simulink model "SingleVehicle_01"  (Simulink 8.8)
settings: Solver=VariableStepAuto  StartTime=0.0  StopTime=35  RelTol=1e-3
undefined symbols (not defined in the file or in its folder): ConnectedBus, DiscIntNeverNeededParam, FromPrescan, IdealSensors, psi, x, y
undefined symbols (not defined in the file): vd
libraries: robotlib x4, PreScanUsefulBlocks x1, PreScanSimulinkLibrary x1
(part 2 of 3)

== matlab function SingleVehicle_01/Controller/CtlMainBusUnitDelayAndInit/MATLAB Function ==
  data: u input double; y output Bus: ControllerMainBus; veh_struct parameter double
function y = DelayAndInitCtlBus(u, veh_struct)
coder.extrinsic('exist')
persistent a

y0 = struct;
y0.ActuationCmdBus = struct;



y0.ActuationCmdBus.steering_cmd = 0;
y0.ActuationCmdBus.decel_cmd = 0;
y0.ActuationCmdBus.accel_cmd = 0;

y0.ArbitratedActuationReq = struct;
y0.ArbitratedActuationReq.v_des = 0;
y0.ArbitratedActuationReq.a_des = 0;
y0.ArbitratedActuationReq.psi_des = 0;
y0.ArbitratedActuationReq.dpsi_des = 0;

y0.FunctionFeatures = struct;
y0.FunctionFeatures.wpFollower = struct;
y0.FunctionFeatures.wpFollower.v_des = 0;
y0.FunctionFeatures.wpFollower.a_des = 0;
y0.FunctionFeatures.wpFollower.psi_des = 0;
y0.FunctionFeatures.wpFollower.dpsi_des = 0;

y0.situationBus = struct;
y0.situationBus.ContextualAwarenessBus = struct;
ObjectBus = struct;
ObjectBus.x = 0;
ObjectBus.y = 0;
ObjectBus.yaw = 0;
y0.situationBus.ContextualAwarenessBus.ObjectsBus = repmat(ObjectBus,100,1);
y0.situationBus.ContextualAwarenessBus.NumberObjects = 10;

y0.situationBus.wP = struct;
y0.situationBus.wP.finalWayPoint = struct;
y0.situationBus.wP.finalWayPoint.x = 0;
y0.situationBus.wP.finalWayPoint.y = 0;
y0.situationBus.wP.finalWayPoint.z = 0;
y0.situationBus.wP.finalWayPoint.treach = 0;

y0.situationBus.wP.currentWayPoint = struct;
y0.situationBus.wP.currentWayPoint.x = 0;
y0.situationBus.wP.currentWayPoint.y = 0;
y0.situationBus.wP.currentWayPoint.z = 0;
y0.situationBus.wP.currentWayPoint.treach = 0;

y0.situationBus.wP.finalWayPointIndex = uint16(1);
y0.situationBus.wP.currentWayPointIndex = uint16(10);

%y0.situationBus.wP.wayPointArray = struct;
wPArray = struct;
wPArray.x = 0;
wPArray.y = 0;
wPArray.z = 0;
wPArray.treach = 0;
y0.situationBus.wP.wayPointArray = repmat(wPArray,100,1);


y0.situationBus.selfAwarenessBus = struct;
y0.situationBus.selfAwarenessBus.x = 0;
y0.situationBus.selfAwarenessBus.y = 0;
y0.situationBus.selfAwarenessBus.z = 0;
y0.situationBus.selfAwarenessBus.theta = 0;
y0.situationBus.selfAwarenessBus.phi = 0;
y0.situationBus.selfAwarenessBus.psi = 0;
y0.situationBus.selfAwarenessBus.u = 0;
y0.situationBus.selfAwarenessBus.v = 0;
y0.situationBus.selfAwarenessBus.w = 0;
y0.situationBus.selfAwarenessBus.dtheta = 0;
y0.situationBus.selfAwarenessBus.dphi = 0;
y0.situationBus.selfAwarenessBus.dpsi = 0;

y0.IdealSensors = struct;
y0.IdealSensors.x = 0;
y0.IdealSensors.y = 0;
y0.IdealSensors.z = 0;
y0.IdealSensors.theta = 0;
y0.IdealSensors.phi = 0;
y0.IdealSensors.psi = 0;
y0.IdealSensors.u = 0;
y0.IdealSensors.v = 0;
y0.IdealSensors.w = 0;
y0.IdealSensors.dtheta = 0;
y0.IdealSensors.dphi = 0;
y0.IdealSensors.dpsi = 0;

y0.FromPrescan = struct;
y0.FromPrescan.x = 0;
y0.FromPrescan.y = 0;
y0.FromPrescan.z = 0;
y0.FromPrescan.Rotx = 0;
y0.FromPrescan.Roty = 0;
y0.FromPrescan.Rotz = 0;
y0.FromPrescan.GPS_lat = 0;
y0.FromPrescan.GPS_long = 0;
y0.FromPrescan.u = 0;
y0.FromPrescan.GPS_alt = 0;
y0.FromPrescan.heading = 0;
y0.FromPrescan.Yaw_rate = 0;


y0.ConnectedBus = struct;
ObjectBus.x = 0;
ObjectBus.y = 0;
ObjectBus.yaw = 0;
y0.ConnectedBus.ObjectsBus = repmat(ObjectBus,100,1);
y0.ConnectedBus.NumberObjects = 10;

% y1 = struct;
% y1.ActuationCmdBus = struct;
% y1.ArbitratedActuationReq = struct;
% y1.FunctionFeatures = struct;
% y1.situationBus = struct;
% y1.situationBus.situationAwarenessBus = struct;
% y1.situationBus.ContextualAwarenessBus = struct;
% y1.situationBus.wP = struct;
% y1.situationBus.wP.finalWayPoint = struct;
% y1.situationBus.wP.currentWayPoint = struct;
% y1.situationBus.selfAwarenessBus = struct;
% 
% 
% y1.ActuationCmdBus.steering_cmd = 0;
% y1.ActuationCmdBus.decel_cmd = 0;
% y1.ActuationCmdBus.accel_cmd = 0;
% 
% y1.ArbitratedActuationReq.v_des = 0;
% y1.ArbitratedActuationReq.a_des = 0;
% y1.ArbitratedActuationReq.psi_des = 0;
% y1.ArbitratedActuationReq.dpsi_des = 0;
% 
% y1.FunctionFeatures.wpFollower = struct;
% y1.FunctionFeatures.wpFollower.v_des = 0;
% y1.FunctionFeatures.wpFollower.a_des = 0;
% y1.FunctionFeatures.wpFollower.psi_des = 0;
% y1.FunctionFeatures.wpFollower.dpsi_des = 0;
% 
% %y1.situationBus.ContextualAwarenessBus.ObjectsBus = struct;
% ObjectBus = struct;
% ObjectBus.x = 0;
% ObjectBus.y = 0;
% ObjectBus.yaw = 0;
% 
% y1.situationBus.ContextualAwarenessBus.ObjectsBus = repmat(ObjectBus,100,1);
% y1.situationBus.ContextualAwarenessBus.ObjectsBus(1, 1).x = 0;
% y1.situationBus.ContextualAwarenessBus.ObjectsBus(1, 1).y = 0;
% y1.situationBus.ContextualAwarenessBus.ObjectsBus(1, 1).yaw = 0;
% y1.situationBus.ContextualAwarenessBus.ObjectsBus(2, 1).x = 0;
% y1.situationBus.ContextualAwarenessBus.ObjectsBus(2, 1).y = 0;
% y1.situationBus.ContextualAwarenessBus.ObjectsBus(2, 1).yaw = 0;
% y1.situationBus.ContextualAwarenessBus.ObjectsBus(3, 1).x = 0;
% y1.situationBus.ContextualAwarenessBus.ObjectsBus(3, 1).y = 0;
% y1.situationBus.ContextualAwarenessBus.ObjectsBus(3, 1).yaw = 0;
% y1.situationBus.ContextualAwarenessBus.ObjectsBus(4, 1).x = 0;
% y1.situationBus.ContextualAwarenessBus.ObjectsBus(4, 1).y = 0;
% y1.situationBus.ContextualAwarenessBus.ObjectsBus(4, 1).yaw = 0;
% y1.situationBus.ContextualAwarenessBus.ObjectsBus(5, 1).x = 0;
% y1.situationBus.ContextualAwarenessBus.ObjectsBus(5, 1).y = 0;
% y1.situationBus.ContextualAwarenessBus.ObjectsBus(5, 1).yaw = 0;
% y1.situationBus.ContextualAwarenessBus.ObjectsBus(6, 1).x = 0;
% y1.situationBus.ContextualAwarenessBus.ObjectsBus(6, 1).y = 0;
% y1.situationBus.ContextualAwarenessBus.ObjectsBus(6, 1).yaw = 0;
% y1.situationBus.ContextualAwarenessBus.ObjectsBus(7, 1).x = 0;
% y1.situationBus.ContextualAwarenessBus.ObjectsBus(7, 1).y = 0;
% y1.situationBus.ContextualAwarenessBus.ObjectsBus(7, 1).yaw = 0;
% y1.situationBus.ContextualAwarenessBus.ObjectsBus(8, 1).x = 0;
% y1.situationBus.ContextualAwarenessBus.ObjectsBus(8, 1).y = 0;
% y1.situationBus.ContextualAwarenessBus.ObjectsBus(8, 1).yaw = 0;
% y1.situationBus.ContextualAwarenessBus.ObjectsBus(9, 1).x = 0;
% y1.situationBus.ContextualAwarenessBus.ObjectsBus(9, 1).y = 0;
% y1.situationBus.ContextualAwarenessBus.ObjectsBus(9, 1).yaw = 0;
% y1.situationBus.ContextualAwarenessBus.ObjectsBus(10, 1).x = 0;
% y1.situationBus.ContextualAwarenessBus.ObjectsBus(10, 1).y = 0;
% y1.situationBus.ContextualAwarenessBus.ObjectsBus(10, 1).yaw = 0;
% y1.situationBus.ContextualAwarenessBus.ObjectsBus(11, 1).x = 0;
% y1.situationBus.ContextualAwarenessBus.ObjectsBus(11, 1).y = 0;
% y1.situationBus.ContextualAwarenessBus.ObjectsBus(11, 1).yaw = 0;
% y1.situationBus.ContextualAwarenessBus.ObjectsBus(12, 1).x = 0;
% y1.situationBus.ContextualAwarenessBus.ObjectsBus(12, 1).y = 0;
% y1.situationBus.ContextualAwarenessBus.ObjectsBus(12, 1).yaw = 0;
% y1.situationBus.ContextualAwarenessBus.ObjectsBus(13, 1).x = 0;
% y1.situationBus.ContextualAwarenessBus.ObjectsBus(13, 1).y = 0;
% y1.situationBus.ContextualAwarenessBus.ObjectsBus(13, 1).yaw = 0;
% y1.situationBus.ContextualAwarenessBus.ObjectsBus(14, 1).x = 0;
% y1.situationBus.ContextualAwarenessBus.ObjectsBus(14, 1).y = 0;
% y1.situationBus.ContextualAwarenessBus.ObjectsBus(14, 1).yaw = 0;
% y1.situationBus.ContextualAwarenessBus.ObjectsBus(15, 1).x = 0;
% y1.situationBus.ContextualAwarenessBus.ObjectsBus(15, 1).y = 0;
% y1.situationBus.ContextualAwarenessBus.ObjectsBus(15, 1).yaw = 0;
% y1.situationBus.ContextualAwarenessBus.ObjectsBus(16, 1).x = 0;
% y1.situationBus.ContextualAwarenessBus.ObjectsBus(16, 1).y = 0;
% y1.situationBus.ContextualAwarenessBus.ObjectsBus(16, 1).yaw = 0;
% y1.situationBus.ContextualAwarenessBus.ObjectsBus(17, 1).x = 0;
% y1.situationBus.ContextualAwarenessBus.ObjectsBus(17, 1).y = 0;
% y1.situationBus.ContextualAwarenessBus.ObjectsBus(17, 1).yaw = 0;
% y1.situationBus.ContextualAwarenessBus.ObjectsBus(18, 1).x = 0;
% y1.situationBus.ContextualAwarenessBus.ObjectsBus(18, 1).y = 0;
% y1.situationBus.ContextualAwarenessBus.ObjectsBus(18, 1).yaw = 0;
% y1.situationBus.ContextualAwarenessBus.ObjectsBus(19, 1).x = 0;
% y1.situationBus.ContextualAwarenessBus.ObjectsBus(19, 1).y = 0;
% y1.situationBus.ContextualAwarenessBus.ObjectsBus(19, 1).yaw = 0;
% y1.situationBus.ContextualAwarenessBus.ObjectsBus(20, 1).x = 0;
% y1.situationBus.ContextualAwarenessBus.ObjectsBus(20, 1).y = 0;
% y1.situationBus.ContextualAwarenessBus.ObjectsBus(20, 1).yaw = 0;
% y1.situationBus.ContextualAwarenessBus.ObjectsBus(21, 1).x = 0;
% y1.situationBus.ContextualAwarenessBus.ObjectsBus(21, 1).y = 0;
% y1.situationBus.ContextualAwarenessBus.ObjectsBus(21, 1).yaw = 0;
% y1.situationBus.ContextualAwarenessBus.ObjectsBus(22, 1).x = 0;
% y1.situationBus.ContextualAwarenessBus.ObjectsBus(22, 1).y = 0;
% y1.situationBus.ContextualAwarenessBus.ObjectsBus(22, 1).yaw = 0;
% y1.situationBus.ContextualAwarenessBus.ObjectsBus(23, 1).x = 0;
% y1.situationBus.ContextualAwarenessBus.ObjectsBus(23, 1).y = 0;
% y1.situationBus.ContextualAwarenessBus.ObjectsBus(23, 1).yaw = 0;
% y1.situationBus.ContextualAwarenessBus.ObjectsBus(24, 1).x = 0;
% y1.situationBus.ContextualAwarenessBus.ObjectsBus(24, 1).y = 0;
% y1.situationBus.ContextualAwarenessBus.ObjectsBus(24, 1).yaw = 0;
% y1.situationBus.ContextualAwarenessBus.ObjectsBus(25, 1).x = 0;
% y1.situationBus.ContextualAwarenessBus.ObjectsBus(25, 1).y = 0;
% y1.situationBus.ContextualAwarenessBus.ObjectsBus(25, 1).yaw = 0;
% y1.situationBus.ContextualAwarenessBus.ObjectsBus(26, 1).x = 0;
% y1.situationBus.ContextualAwarenessBus.ObjectsBus(26, 1).y = 0;
% y1.situationBus.ContextualAwarenessBus.ObjectsBus(26, 1).yaw = 0;
% y1.situationBus.ContextualAwarenessBus.ObjectsBus(27, 1).x = 0;
% y1.situationBus.ContextualAwarenessBus.ObjectsBus(27, 1).y = 0;
% y1.situationBus.ContextualAwarenessBus.ObjectsBus(27, 1).yaw = 0;
% y1.situationBus.ContextualAwarenessBus.ObjectsBus(28, 1).x = 0;
% y1.situationBus.ContextualAwarenessBus.ObjectsBus(28, 1).y = 0;
% y1.situationBus.ContextualAwarenessBus.ObjectsBus(28, 1).yaw = 0;
% y1.situationBus.ContextualAwarenessBus.ObjectsBus(29, 1).x = 0;
% y1.situationBus.ContextualAwarenessBus.ObjectsBus(29, 1).y = 0;
% y1.situationBus.ContextualAwarenessBus.ObjectsBus(29, 1).yaw = 0;
% y1.situationBus.ContextualAwarenessBus.ObjectsBus(30, 1).x = 0;
% y1.situationBus.ContextualAwarenessBus.ObjectsBus(30, 1).y = 0;
% y1.situationBus.ContextualAwarenessBus.ObjectsBus(30, 1).yaw = 0;
% y1.situationBus.ContextualAwarenessBus.ObjectsBus(31, 1).x = 0;
% y1.situationBus.ContextualAwarenessBus.ObjectsBus(31, 1).y = 0;
% y1.situationBus.ContextualAwarenessBus.ObjectsBus(31, 1).yaw = 0;
% y1.situationBus.ContextualAwarenessBus.ObjectsBus(32, 1).x = 0;
% y1.situationBus.ContextualAwarenessBus.ObjectsBus(32, 1).y = 0;
% y1.situationBus.ContextualAwarenessBus.ObjectsBus(32, 1).yaw = 0;
% y1.situationBus.ContextualAwarenessBus.ObjectsBus(33, 1).x = 0;
% y1.situationBus.ContextualAwarenessBus.ObjectsBus(33, 1).y = 0;
% y1.situationBus.ContextualAwarenessBus.ObjectsBus(33, 1).yaw = 0;
% y1.situationBus.ContextualAwarenessBus.ObjectsBus(34, 1).x = 0;
% y1.situationBus.ContextualAwarenessBus.ObjectsBus(34, 1).y = 0;
% y1.situationBus.ContextualAwarenessBus.ObjectsBus(34, 1).yaw = 0;
% y1.situationBus.ContextualAwarenessBus.ObjectsBus(35, 1).x = 0;
% y1.situationBus.ContextualAwarenessBus.ObjectsBus(35, 1).y = 0;
% y1.situationBus.ContextualAwarenessBus.ObjectsBus(35, 1).yaw = 0;
% y1.situationBus.ContextualAwarenessBus.ObjectsBus(36, 1).x = 0;
% y1.situationBus.ContextualAwarenessBus.ObjectsBus(36, 1).y = 0;
% y1.situationBus.ContextualAwarenessBus.ObjectsBus(36, 1).yaw = 0;
% y1.situationBus.ContextualAwarenessBus.ObjectsBus(37, 1).x = 0;
% y1.situationBus.ContextualAwarenessBus.ObjectsBus(37, 1).y = 0;
% y1.situationBus.ContextualAwarenessBus.ObjectsBus(37, 1).yaw = 0;
% y1.situationBus.ContextualAwarenessBus.ObjectsBus(38, 1).x = 0;
% y1.situationBus.ContextualAwarenessBus.ObjectsBus(38, 1).y = 0;
% y1.situationBus.ContextualAwarenessBus.ObjectsBus(38, 1).yaw = 0;
% y1.situationBus.ContextualAwarenessBus.ObjectsBus(39, 1).x = 0;
% y1.situationBus.ContextualAwarenessBus.ObjectsBus(39, 1).y = 0;
% y1.situationBus.ContextualAwarenessBus.ObjectsBus(39, 1).yaw = 0;
% y1.situationBus.ContextualAwarenessBus.ObjectsBus(40, 1).x = 0;
% y1.situationBus.ContextualAwarenessBus.ObjectsBus(40, 1).y = 0;
% y1.situationBus.ContextualAwarenessBus.ObjectsBus(40, 1).yaw = 0;
% y1.situationBus.ContextualAwarenessBus.ObjectsBus(41, 1).x = 0;
% y1.situationBus.ContextualAwarenessBus.ObjectsBus(41, 1).y = 0;
% y1.situationBus.ContextualAwarenessBus.ObjectsBus(41, 1).yaw = 0;
% y1.situationBus.ContextualAwarenessBus.ObjectsBus(42, 1).x = 0;
% y1.situationBus.ContextualAwarenessBus.ObjectsBus(42, 1).y = 0;
% y1.situationBus.ContextualAwarenessBus.ObjectsBus(42, 1).yaw = 0;
% y1.situationBus.ContextualAwarenessBus.ObjectsBus(43, 1).x = 0;
% y1.situationBus.ContextualAwarenessBus.ObjectsBus(43, 1).y = 0;
% y1.situationBus.ContextualAwarenessBus.ObjectsBus(43, 1).yaw = 0;
% y1.situationBus.ContextualAwarenessBus.ObjectsBus(44, 1).x = 0;
% y1.situationBus.ContextualAwarenessBus.ObjectsBus(44, 1).y = 0;
% y1.situationBus.ContextualAwarenessBus.ObjectsBus(44, 1).yaw = 0;
% y1.situationBus.ContextualAwarenessBus.ObjectsBus(45, 1).x = 0;
% y1.situationBus.ContextualAwarenessBus.ObjectsBus(45, 1).y = 0;
% y1.situationBus.ContextualAwarenessBus.ObjectsBus(45, 1).yaw = 0;
% y1.situationBus.ContextualAwarenessBus.ObjectsBus(46, 1).x = 0;
% y1.situationBus.ContextualAwarenessBus.ObjectsBus(46, 1).y = 0;
% y1.situationBus.ContextualAwarenessBus.ObjectsBus(46, 1).yaw = 0;
% y1.situationBus.ContextualAwarenessBus.ObjectsBus(47, 1).x = 0;
% y1.situationBus.ContextualAwarenessBus.ObjectsBus(47, 1).y = 0;
% y1.situationBus.ContextualAwarenessBus.ObjectsBus(47, 1).yaw = 0;
% y1.situationBus.ContextualAwarenessBus.ObjectsBus(48, 1).x = 0;
% y1.situationBus.ContextualAwarenessBus.ObjectsBus(48, 1).y = 0;
% y1.situationBus.ContextualAwarenessBus.ObjectsBus(48, 1).yaw = 0;
% y1.situationBus.ContextualAwarenessBus.ObjectsBus(49, 1).x = 0;
% y1.situationBus.ContextualAwarenessBus.ObjectsBus(49, 1).y = 0;
% y1.situationBus.ContextualAwarenessBus.ObjectsBus(49, 1).yaw = 0;
% y1.situationBus.ContextualAwarenessBus.ObjectsBus(50, 1).x = 0;
% y1.situationBus.ContextualAwarenessBus.ObjectsBus(50, 1).y = 0;
% y1.situationBus.ContextualAwarenessBus.ObjectsBus(50, 1).yaw = 0;
% y1.situationBus.ContextualAwarenessBus.ObjectsBus(51, 1).x = 0;
% y1.situationBus.ContextualAwarenessBus.ObjectsBus(51, 1).y = 0;
% y1.situationBus.ContextualAwarenessBus.ObjectsBus(51, 1).yaw = 0;
% y1.situationBus.ContextualAwarenessBus.ObjectsBus(52, 1).x = 0;
% y1.situationBus.ContextualAwarenessBus.ObjectsBus(52, 1).y = 0;
% y1.situationBus.ContextualAwarenessBus.ObjectsBus(52, 1).yaw = 0;
% y1.situationBus.ContextualAwarenessBus.ObjectsBus(53, 1).x = 0;
% y1.situationBus.ContextualAwarenessBus.ObjectsBus(53, 1).y = 0;
% y1.situationBus.ContextualAwarenessBus.ObjectsBus(53, 1).yaw = 0;
% y1.situationBus.ContextualAwarenessBus.ObjectsBus(54, 1).x = 0;
% y1.situationBus.ContextualAwarenessBus.ObjectsBus(54, 1).y = 0;
% y1.situationBus.ContextualAwarenessBus.ObjectsBus(54, 1).yaw = 0;
% y1.situationBus.ContextualAwarenessBus.ObjectsBus(55, 1).x = 0;
% y1.situationBus.ContextualAwarenessBus.ObjectsBus(55, 1).y = 0;
% y1.situationBus.ContextualAwarenessBus.ObjectsBus(55, 1).yaw = 0;
% y1.situationBus.ContextualAwarenessBus.ObjectsBus(56, 1).x = 0;
% y1.situationBus.ContextualAwarenessBus.ObjectsBus(56, 1).y = 0;
% y1.situationBus.ContextualAwarenessBus.ObjectsBus(56, 1).yaw = 0;
% y1.situationBus.ContextualAwarenessBus.ObjectsBus(57, 1).x = 0;
% y1.situationBus.ContextualAwarenessBus.ObjectsBus(57, 1).y = 0;
% y1.situationBus.ContextualAwarenessBus.ObjectsBus(57, 1).yaw = 0;
% y1.situationBus.ContextualAwarenessBus.ObjectsBus(58, 1).x = 0;
% y1.situationBus.ContextualAwarenessBus.ObjectsBus(58, 1).y = 0;
% y1.situationBus.ContextualAwarenessBus.ObjectsBus(58, 1).yaw = 0;
% y1.situationBus.ContextualAwarenessBus.ObjectsBus(59, 1).x = 0;
% y1.situationBus.ContextualAwarenessBus.ObjectsBus(59, 1).y = 0;
% y1.situationBus.ContextualAwarenessBus.ObjectsBus(59, 1).yaw = 0;
% y1.situationBus.ContextualAwarenessBus.ObjectsBus(60, 1).x = 0;
% y1.situationBus.ContextualAwarenessBus.ObjectsBus(60, 1).y = 0;
% y1.situationBus.ContextualAwarenessBus.ObjectsBus(60, 1).yaw = 0;
% y1.situationBus.ContextualAwarenessBus.ObjectsBus(61, 1).x = 0;
% y1.situationBus.ContextualAwarenessBus.ObjectsBus(61, 1).y = 0;
% y1.situationBus.ContextualAwarenessBus.ObjectsBus(61, 1).yaw = 0;
% y1.situationBus.ContextualAwarenessBus.ObjectsBus(62, 1).x = 0;
% y1.situationBus.ContextualAwarenessBus.ObjectsBus(62, 1).y = 0;
% y1.situationBus.ContextualAwarenessBus.ObjectsBus(62, 1).yaw = 0;
% y1.situationBus.ContextualAwarenessBus.ObjectsBus(63, 1).x = 0;
% y1.situationBus.ContextualAwarenessBus.ObjectsBus(63, 1).y = 0;
% y1.situationBus.ContextualAwarenessBus.ObjectsBus(63, 1).yaw = 0;
% y1.situationBus.ContextualAwarenessBus.ObjectsBus(64, 1).x = 0;
% y1.situationBus.ContextualAwarenessBus.ObjectsBus(64, 1).y = 0;
% y1.situationBus.ContextualAwarenessBus.ObjectsBus(64, 1).yaw = 0;
% y1.situationBus.ContextualAwarenessBus.ObjectsBus(65, 1).x = 0;
% y1.situationBus.ContextualAwarenessBus.ObjectsBus(65, 1).y = 0;
% y1.situationBus.ContextualAwarenessBus.ObjectsBus(65, 1).yaw = 0;
% y1.situationBus.ContextualAwarenessBus.ObjectsBus(66, 1).x = 0;
% y1.situationBus.ContextualAwarenessBus.ObjectsBus(66, 1).y = 0;
% y1.situationBus.ContextualAwarenessBus.ObjectsBus(66, 1).yaw = 0;
% y1.situationBus.ContextualAwarenessBus.ObjectsBus(67, 1).x = 0;
% y1.situationBus.ContextualAwarenessBus.ObjectsBus(67, 1).y = 0;
% y1.situationBus.ContextualAwarenessBus.ObjectsBus(67, 1).yaw = 0;
% y1.situationBus.ContextualAwarenessBus.ObjectsBus(68, 1).x = 0;
% y1.situationBus.ContextualAwarenessBus.ObjectsBus(68, 1).y = 0;
% y1.situationBus.ContextualAwarenessBus.ObjectsBus(68, 1).yaw = 0;
% y1.situationBus.ContextualAwarenessBus.ObjectsBus(69, 1).x = 0;
% y1.situationBus.ContextualAwarenessBus.ObjectsBus(69, 1).y = 0;
% y1.situationBus.ContextualAwarenessBus.ObjectsBus(69, 1).yaw = 0;
% y1.situationBus.ContextualAwarenessBus.ObjectsBus(70, 1).x = 0;
% y1.situationBus.ContextualAwarenessBus.ObjectsBus(70, 1).y = 0;
% y1.situationBus.ContextualAwarenessBus.ObjectsBus(70, 1).yaw = 0;
% y1.situationBus.ContextualAwarenessBus.ObjectsBus(71, 1).x = 0;
% y1.situationBus.ContextualAwarenessBus.ObjectsBus(71, 1).y = 0;
% y1.situationBus.ContextualAwarenessBus.ObjectsBus(71, 1).yaw = 0;
% y1.situationBus.ContextualAwarenessBus.ObjectsBus(72, 1).x = 0;
% y1.situationBus.ContextualAwarenessBus.ObjectsBus(72, 1).y = 0;
% y1.situationBus.ContextualAwarenessBus.ObjectsBus(72, 1).yaw = 0;
% y1.situationBus.ContextualAwarenessBus.ObjectsBus(73, 1).x = 0;
% y1.situationBus.ContextualAwarenessBus.ObjectsBus(73, 1).y = 0;
% y1.situationBus.ContextualAwarenessBus.ObjectsBus(73, 1).yaw = 0;
% y1.situationBus.ContextualAwarenessBus.ObjectsBus(74, 1).x = 0;
% y1.situationBus.ContextualAwarenessBus.ObjectsBus(74, 1).y = 0;
% y1.situationBus.ContextualAwarenessBus.ObjectsBus(74, 1).yaw = 0;
% y1.situationBus.ContextualAwarenessBus.ObjectsBus(75, 1).x = 0;
% y1.situationBus.ContextualAwarenessBus.ObjectsBus(75, 1).y = 0;
% y1.situationBus.ContextualAwarenessBus.ObjectsBus(75, 1).yaw = 0;
% y1.situationBus.ContextualAwarenessBus.ObjectsBus(76, 1).x = 0;
% y1.situationBus.ContextualAwarenessBus.ObjectsBus(76, 1).y = 0;
% y1.situationBus.ContextualAwarenessBus.ObjectsBus(76, 1).yaw = 0;
% y1.situationBus.ContextualAwarenessBus.ObjectsBus(77, 1).x = 0;
% y1.situationBus.ContextualAwarenessBus.ObjectsBus(77, 1).y = 0;
% y1.situationBus.ContextualAwarenessBus.ObjectsBus(77, 1).yaw = 0;
% y1.situationBus.ContextualAwarenessBus.ObjectsBus(78, 1).x = 0;
% y1.situationBus.ContextualAwarenessBus.ObjectsBus(78, 1).y = 0;
% y1.situationBus.ContextualAwarenessBus.ObjectsBus(78, 1).yaw = 0;
% y1.situationBus.ContextualAwarenessBus.ObjectsBus(79, 1).x = 0;
% y1.situationBus.ContextualAwarenessBus.ObjectsBus(79, 1).y = 0;
% y1.situationBus.ContextualAwarenessBus.ObjectsBus(79, 1).yaw = 0;
% y1.situationBus.ContextualAwarenessBus.ObjectsBus(80, 1).x = 0;
% y1.situationBus.ContextualAwarenessBus.ObjectsBus(80, 1).y = 0;
% y1.situationBus.ContextualAwarenessBus.ObjectsBus(80, 1).yaw = 0;
% y1.situationBus.ContextualAwarenessBus.ObjectsBus(81, 1).x = 0;
% y1.situationBus.ContextualAwarenessBus.ObjectsBus(81, 1).y = 0;
% y1.situationBus.ContextualAwarenessBus.ObjectsBus(81, 1).yaw = 0;
% y1.situationBus.ContextualAwarenessBus.ObjectsBus(82, 1).x = 0;
% y1.situationBus.ContextualAwarenessBus.ObjectsBus(82, 1).y = 0;
% y1.situationBus.ContextualAwarenessBus.ObjectsBus(82, 1).yaw = 0;
% y1.situationBus.ContextualAwarenessBus.ObjectsBus(83, 1).x = 0;
% y1.situationBus.ContextualAwarenessBus.ObjectsBus(83, 1).y = 0;
% y1.situationBus.ContextualAwarenessBus.ObjectsBus(83, 1).yaw = 0;
% y1.situationBus.ContextualAwarenessBus.ObjectsBus(84, 1).x = 0;
% y1.situationBus.ContextualAwarenessBus.ObjectsBus(84, 1).y = 0;
% y1.situationBus.ContextualAwarenessBus.ObjectsBus(84, 1).yaw = 0;
% y1.situationBus.ContextualAwarenessBus.ObjectsBus(85, 1).x = 0;
% y1.situationBus.ContextualAwarenessBus.ObjectsBus(85, 1).y = 0;
% y1.situationBus.ContextualAwarenessBus.ObjectsBus(85, 1).yaw = 0;
% y1.situationBus.ContextualAwarenessBus.ObjectsBus(86, 1).x = 0;
% y1.situationBus.ContextualAwarenessBus.ObjectsBus(86, 1).y = 0;
% y1.situationBus.ContextualAwarenessBus.ObjectsBus(86, 1).yaw = 0;
% y1.situationBus.ContextualAwarenessBus.ObjectsBus(87, 1).x = 0;
% y1.situationBus.ContextualAwarenessBus.ObjectsBus(87, 1).y = 0;
% y1.situationBus.ContextualAwarenessBus.ObjectsBus(87, 1).yaw = 0;
% y1.situationBus.ContextualAwarenessBus.ObjectsBus(88, 1).x = 0;
% y1.situationBus.ContextualAwarenessBus.ObjectsBus(88, 1).y = 0;
% y1.situationBus.ContextualAwarenessBus.ObjectsBus(88, 1).yaw = 0;
% y1.situationBus.ContextualAwarenessBus.ObjectsBus(89, 1).x = 0;
% y1.situationBus.ContextualAwarenessBus.ObjectsBus(89, 1).y = 0;
% y1.situationBus.ContextualAwarenessBus.ObjectsBus(89, 1).yaw = 0;
% y1.situationBus.ContextualAwarenessBus.ObjectsBus(90, 1).x = 0;
% y1.situationBus.ContextualAwarenessBus.ObjectsBus(90, 1).y = 0;
% y1.situationBus.ContextualAwarenessBus.ObjectsBus(90, 1).yaw = 0;
% y1.situationBus.ContextualAwarenessBus.ObjectsBus(91, 1).x = 0;
% y1.situationBus.ContextualAwarenessBus.ObjectsBus(91, 1).y = 0;
% y1.situationBus.ContextualAwarenessBus.ObjectsBus(91, 1).yaw = 0;
% y1.situationBus.ContextualAwarenessBus.ObjectsBus(92, 1).x = 0;
% y1.situationBus.ContextualAwarenessBus.ObjectsBus(92, 1).y = 0;
% y1.situationBus.ContextualAwarenessBus.ObjectsBus(92, 1).yaw = 0;
% y1.situationBus.ContextualAwarenessBus.ObjectsBus(93, 1).x = 0;
% y1.situationBus.ContextualAwarenessBus.ObjectsBus(93, 1).y = 0;
% y1.situationBus.ContextualAwarenessBus.ObjectsBus(93, 1).yaw = 0;
% y1.situationBus.ContextualAwarenessBus.ObjectsBus(94, 1).x = 0;
% y1.situationBus.ContextualAwarenessBus.ObjectsBus(94, 1).y = 0;
% y1.situationBus.ContextualAwarenessBus.ObjectsBus(94, 1).yaw = 0;
% y1.situationBus.ContextualAwarenessBus.ObjectsBus(95, 1).x = 0;
% y1.situationBus.ContextualAwarenessBus.ObjectsBus(95, 1).y = 0;
% y1.situationBus.ContextualAwarenessBus.ObjectsBus(95, 1).yaw = 0;
% y1.situationBus.ContextualAwarenessBus.ObjectsBus(96, 1).x = 0;
% y1.situationBus.ContextualAwarenessBus.ObjectsBus(96, 1).y = 0;
% y1.situationBus.ContextualAwarenessBus.ObjectsBus(96, 1).yaw = 0;
% y1.situationBus.ContextualAwarenessBus.ObjectsBus(97, 1).x = 0;
% y1.situationBus.ContextualAwarenessBus.ObjectsBus(97, 1).y = 0;
% y1.situationBus.ContextualAwarenessBus.ObjectsBus(97, 1).yaw = 0;
% y1.situationBus.ContextualAwarenessBus.ObjectsBus(98, 1).x = 0;
% y1.situationBus.ContextualAwarenessBus.ObjectsBus(98, 1).y = 0;
% y1.situationBus.ContextualAwarenessBus.ObjectsBus(98, 1).yaw = 0;
% y1.situationBus.ContextualAwarenessBus.ObjectsBus(99, 1).x = 0;
% y1.situationBus.ContextualAwarenessBus.ObjectsBus(99, 1).y = 0;
% y1.situationBus.ContextualAwarenessBus.ObjectsBus(99, 1).yaw = 0;
% y1.situationBus.ContextualAwarenessBus.ObjectsBus(100, 1).x = 0;
% y1.situationBus.ContextualAwarenessBus.ObjectsBus(100, 1).y = 0;
% y1.situationBus.ContextualAwarenessBus.ObjectsBus(100, 1).yaw = 0;
% y1.situationBus.ContextualAwarenessBus.NumberObjects = 0;
% 
% y1.situationBus.wP.finalWayPoint.x = 0;
% y1.situationBus.wP.finalWayPoint.y = 0;
% y1.situationBus.wP.finalWayPoint.z = 0;
% y1.situationBus.wP.finalWayPoint.treach = 0;
% 
% y1.situationBus.wP.currentWayPoint.x = 0;
% y1.situationBus.wP.currentWayPoint.y = 0;
% y1.situationBus.wP.currentWayPoint.z = 0;
% y1.situationBus.wP.currentWayPoint.treach = 0;
% y1.situationBus.wP.finalWayPointIndex = uint16(0);
% y1.situationBus.wP.currentWayPointIndex = uint16(0);
% %y1.situationBus.wP.wayPointArray = struct;
% wPpoint = struct;
% wPpoint.x = 0;
% wPpoint.y = 0;
% wPpoint.z = 0;
% wPpoint.treach = 0;
% y1.situationBus.wP.wayPointArray = repmat(wPpoint,100,1)
% y1.situationBus.wP.wayPointArray(1, 1).x = 0;
% y1.situationBus.wP.wayPointArray(1, 1).y = 0;
% y1.situationBus.wP.wayPointArray(1, 1).z = 0;
% y1.situationBus.wP.wayPointArray(1, 1).treach = 0;
% y1.situationBus.wP.wayPointArray(2, 1).x = 0;
% y1.situationBus.wP.wayPointArray(2, 1).y = 0;
% y1.situationBus.wP.wayPointArray(2, 1).z = 0;
% y1.situationBus.wP.wayPointArray(2, 1).treach = 0;
% y1.situationBus.wP.wayPointArray(3, 1).x = 0;
% y1.situationBus.wP.wayPointArray(3, 1).y = 0;
% y1.situationBus.wP.wayPointArray(3, 1).z = 0;
% y1.situationBus.wP.wayPointArray(3, 1).treach = 0;
% y1.situationBus.wP.wayPointArray(4, 1).x = 0;
% y1.situationBus.wP.wayPointArray(4, 1).y = 0;
% y1.situationBus.wP.wayPointArray(4, 1).z = 0;
% y1.situationBus.wP.wayPointArray(4, 1).treach = 0;
% y1.situationBus.wP.wayPointArray(5, 1).x = 0;
% y1.situationBus.wP.wayPointArray(5, 1).y = 0;
% y1.situationBus.wP.wayPointArray(5, 1).z = 0;
% y1.situationBus.wP.wayPointArray(5, 1).treach = 0;
% y1.situationBus.wP.wayPointArray(6, 1).x = 0;
% y1.situationBus.wP.wayPointArray(6, 1).y = 0;
% y1.situationBus.wP.wayPointArray(6, 1).z = 0;
% y1.situationBus.wP.wayPointArray(6, 1).treach = 0;
% y1.situationBus.wP.wayPointArray(7, 1).x = 0;
% y1.situationBus.wP.wayPointArray(7, 1).y = 0;
% y1.situationBus.wP.wayPointArray(7, 1).z = 0;
% y1.situationBus.wP.wayPointArray(7, 1).treach = 0;
% y1.situationBus.wP.wayPointArray(8, 1).x = 0;
% y1.situationBus.wP.wayPointArray(8, 1).y = 0;
% y1.situationBus.wP.wayPointArray(8, 1).z = 0;
% y1.situationBus.wP.wayPointArray(8, 1).treach = 0;
% y1.situationBus.wP.wayPointArray(9, 1).x = 0;
% y1.situationBus.wP.wayPointArray(9, 1).y = 0;
% y1.situationBus.wP.wayPointArray(9, 1).z = 0;
% y1.situationBus.wP.wayPointArray(9, 1).treach = 0;
% y1.situationBus.wP.wayPointArray(10, 1).x = 0;
% y1.situationBus.wP.wayPointArray(10, 1).y = 0;
% y1.situationBus.wP.wayPointArray(10, 1).z = 0;
% y1.situationBus.wP.wayPointArray(10, 1).treach = 0;
% y1.situationBus.wP.wayPointArray(11, 1).x = 0;
% y1.situationBus.wP.wayPointArray(11, 1).y = 0;
% y1.situationBus.wP.wayPointArray(11, 1).z = 0;
% y1.situationBus.wP.wayPointArray(11, 1).treach = 0;
% y1.situationBus.wP.wayPointArray(12, 1).x = 0;
% y1.situationBus.wP.wayPointArray(12, 1).y = 0;
% y1.situationBus.wP.wayPointArray(12, 1).z = 0;
% y1.situationBus.wP.wayPointArray(12, 1).treach = 0;
% y1.situationBus.wP.wayPointArray(13, 1).x = 0;
% y1.situationBus.wP.wayPointArray(13, 1).y = 0;
% y1.situationBus.wP.wayPointArray(13, 1).z = 0;
% y1.situationBus.wP.wayPointArray(13, 1).treach = 0;
% y1.situationBus.wP.wayPointArray(14, 1).x = 0;
% y1.situationBus.wP.wayPointArray(14, 1).y = 0;
% y1.situationBus.wP.wayPointArray(14, 1).z = 0;
% y1.situationBus.wP.wayPointArray(14, 1).treach = 0;
% y1.situationBus.wP.wayPointArray(15, 1).x = 0;
% y1.situationBus.wP.wayPointArray(15, 1).y = 0;
% y1.situationBus.wP.wayPointArray(15, 1).z = 0;
% y1.situationBus.wP.wayPointArray(15, 1).treach = 0;
% y1.situationBus.wP.wayPointArray(16, 1).x = 0;
% y1.situationBus.wP.wayPointArray(16, 1).y = 0;
% y1.situationBus.wP.wayPointArray(16, 1).z = 0;
% y1.situationBus.wP.wayPointArray(16, 1).treach = 0;
% y1.situationBus.wP.wayPointArray(17, 1).x = 0;
% y1.situationBus.wP.wayPointArray(17, 1).y = 0;
% y1.situationBus.wP.wayPointArray(17, 1).z = 0;
% y1.situationBus.wP.wayPointArray(17, 1).treach = 0;
% y1.situationBus.wP.wayPointArray(18, 1).x = 0;
% y1.situationBus.wP.wayPointArray(18, 1).y = 0;
% y1.situationBus.wP.wayPointArray(18, 1).z = 0;
% y1.situationBus.wP.wayPointArray(18, 1).treach = 0;
% y1.situationBus.wP.wayPointArray(19, 1).x = 0;
% y1.situationBus.wP.wayPointArray(19, 1).y = 0;
% y1.situationBus.wP.wayPointArray(19, 1).z = 0;
% y1.situationBus.wP.wayPointArray(19, 1).treach = 0;
% y1.situationBus.wP.wayPointArray(20, 1).x = 0;
% y1.situationBus.wP.wayPointArray(20, 1).y = 0;
% y1.situationBus.wP.wayPointArray(20, 1).z = 0;
% y1.situationBus.wP.wayPointArray(20, 1).treach = 0;
% y1.situationBus.wP.wayPointArray(21, 1).x = 0;
% y1.situationBus.wP.wayPointArray(21, 1).y = 0;
% y1.situationBus.wP.wayPointArray(21, 1).z = 0;
% y1.situationBus.wP.wayPointArray(21, 1).treach = 0;
% y1.situationBus.wP.wayPointArray(22, 1).x = 0;
% y1.situationBus.wP.wayPointArray(22, 1).y = 0;
% y1.situationBus.wP.wayPointArray(22, 1).z = 0;
% y1.situationBus.wP.wayPointArray(22, 1).treach = 0;
% y1.situationBus.wP.wayPointArray(23, 1).x = 0;
% y1.situationBus.wP.wayPointArray(23, 1).y = 0;
% y1.situationBus.wP.wayPointArray(23, 1).z = 0;
% y1.situationBus.wP.wayPointArray(23, 1).treach = 0;
% y1.situationBus.wP.wayPointArray(24, 1).x = 0;
% y1.situationBus.wP.wayPointArray(24, 1).y = 0;
% y1.situationBus.wP.wayPointArray(24, 1).z = 0;
% y1.situationBus.wP.wayPointArray(24, 1).treach = 0;
% y1.situationBus.wP.wayPointArray(25, 1).x = 0;
% y1.situationBus.wP.wayPointArray(25, 1).y = 0;
% y1.situationBus.wP.wayPointArray(25, 1).z = 0;
% y1.situationBus.wP.wayPointArray(25, 1).treach = 0;
% y1.situationBus.wP.wayPointArray(26, 1).x = 0;
% y1.situationBus.wP.wayPointArray(26, 1).y = 0;
% y1.situationBus.wP.wayPointArray(26, 1).z = 0;
% y1.situationBus.wP.wayPointArray(26, 1).treach = 0;
% y1.situationBus.wP.wayPointArray(27, 1).x = 0;
% y1.situationBus.wP.wayPointArray(27, 1).y = 0;
% y1.situationBus.wP.wayPointArray(27, 1).z = 0;
% y1.situationBus.wP.wayPointArray(27, 1).treach = 0;
% y1.situationBus.wP.wayPointArray(28, 1).x = 0;
% y1.situationBus.wP.wayPointArray(28, 1).y = 0;
% y1.situationBus.wP.wayPointArray(28, 1).z = 0;
% y1.situationBus.wP.wayPointArray(28, 1).treach = 0;
% y1.situationBus.wP.wayPointArray(29, 1).x = 0;
% y1.situationBus.wP.wayPointArray(29, 1).y = 0;
% y1.situationBus.wP.wayPointArray(29, 1).z = 0;
% y1.situationBus.wP.wayPointArray(29, 1).treach = 0;
% y1.situationBus.wP.wayPointArray(30, 1).x = 0;
% y1.situationBus.wP.wayPointArray(30, 1).y = 0;
% y1.situationBus.wP.wayPointArray(30, 1).z = 0;
% y1.situationBus.wP.wayPointArray(30, 1).treach = 0;
% y1.situationBus.wP.wayPointArray(31, 1).x = 0;
% y1.situationBus.wP.wayPointArray(31, 1).y = 0;
% y1.situationBus.wP.wayPointArray(31, 1).z = 0;
% y1.situationBus.wP.wayPointArray(31, 1).treach = 0;
% y1.situationBus.wP.wayPointArray(32, 1).x = 0;
% y1.situationBus.wP.wayPointArray(32, 1).y = 0;
% y1.situationBus.wP.wayPointArray(32, 1).z = 0;
% y1.situationBus.wP.wayPointArray(32, 1).treach = 0;
% y1.situationBus.wP.wayPointArray(33, 1).x = 0;
% y1.situationBus.wP.wayPointArray(33, 1).y = 0;
% y1.situationBus.wP.wayPointArray(33, 1).z = 0;
% y1.situationBus.wP.wayPointArray(33, 1).treach = 0;
% y1.situationBus.wP.wayPointArray(34, 1).x = 0;
% y1.situationBus.wP.wayPointArray(34, 1).y = 0;
% y1.situationBus.wP.wayPointArray(34, 1).z = 0;
% y1.situationBus.wP.wayPointArray(34, 1).treach = 0;
% y1.situationBus.wP.wayPointArray(35, 1).x = 0;
% y1.situationBus.wP.wayPointArray(35, 1).y = 0;
% y1.situationBus.wP.wayPointArray(35, 1).z = 0;
% y1.situationBus.wP.wayPointArray(35, 1).treach = 0;
% y1.situationBus.wP.wayPointArray(36, 1).x = 0;
% y1.situationBus.wP.wayPointArray(36, 1).y = 0;
% y1.situationBus.wP.wayPointArray(36, 1).z = 0;
% y1.situationBus.wP.wayPointArray(36, 1).treach = 0;
% y1.situationBus.wP.wayPointArray(37, 1).x = 0;
% y1.situationBus.wP.wayPointArray(37, 1).y = 0;
% y1.situationBus.wP.wayPointArray(37, 1).z = 0;
% y1.situationBus.wP.wayPointArray(37, 1).treach = 0;
% y1.situationBus.wP.wayPointArray(38, 1).x = 0;
% y1.situationBus.wP.wayPointArray(38, 1).y = 0;
% y1.situationBus.wP.wayPointArray(38, 1).z = 0;
% y1.situationBus.wP.wayPointArray(38, 1).treach = 0;
% y1.situationBus.wP.wayPointArray(39, 1).x = 0;
% y1.situationBus.wP.wayPointArray(39, 1).y = 0;
% y1.situationBus.wP.wayPointArray(39, 1).z = 0;
% y1.situationBus.wP.wayPointArray(39, 1).treach = 0;
% y1.situationBus.wP.wayPointArray(40, 1).x = 0;
% y1.situationBus.wP.wayPointArray(40, 1).y = 0;
% y1.situationBus.wP.wayPointArray(40, 1).z = 0;
% y1.situationBus.wP.wayPointArray(40, 1).treach = 0;
% y1.situationBus.wP.wayPointArray(41, 1).x = 0;
% y1.situationBus.wP.wayPointArray(41, 1).y = 0;
% y1.situationBus.wP.wayPointArray(41, 1).z = 0;
% y1.situationBus.wP.wayPointArray(41, 1).treach = 0;
% y1.situationBus.wP.wayPointArray(42, 1).x = 0;
% y1.situationBus.wP.wayPointArray(42, 1).y = 0;
% y1.situationBus.wP.wayPointArray(42, 1).z = 0;
% y1.situationBus.wP.wayPointArray(42, 1).treach = 0;
% y1.situationBus.wP.wayPointArray(43, 1).x = 0;
% y1.situationBus.wP.wayPointArray(43, 1).y = 0;
% y1.situationBus.wP.wayPointArray(43, 1).z = 0;
% y1.situationBus.wP.wayPointArray(43, 1).treach = 0;
% y1.situationBus.wP.wayPointArray(44, 1).x = 0;
% y1.situationBus.wP.wayPointArray(44, 1).y = 0;
% y1.situationBus.wP.wayPointArray(44, 1).z = 0;
% y1.situationBus.wP.wayPointArray(44, 1).treach = 0;
% y1.situationBus.wP.wayPointArray(45, 1).x = 0;
% y1.situationBus.wP.wayPointArray(45, 1).y = 0;
% y1.situationBus.wP.wayPointArray(45, 1).z = 0;
% y1.situationBus.wP.wayPointArray(45, 1).treach = 0;
% y1.situationBus.wP.wayPointArray(46, 1).x = 0;
% y1.situationBus.wP.wayPointArray(46, 1).y = 0;
% y1.situationBus.wP.wayPointArray(46, 1).z = 0;
% y1.situationBus.wP.wayPointArray(46, 1).treach = 0;
% y1.situationBus.wP.wayPointArray(47, 1).x = 0;
% y1.situationBus.wP.wayPointArray(47, 1).y = 0;
% y1.situationBus.wP.wayPointArray(47, 1).z = 0;
% y1.situationBus.wP.wayPointArray(47, 1).treach = 0;
% y1.situationBus.wP.wayPointArray(48, 1).x = 0;
% y1.situationBus.wP.wayPointArray(48, 1).y = 0;
% y1.situationBus.wP.wayPointArray(48, 1).z = 0;
% y1.situationBus.wP.wayPointArray(48, 1).treach = 0;
% y1.situationBus.wP.wayPointArray(49, 1).x = 0;
% y1.situationBus.wP.wayPointArray(49, 1).y = 0;
% y1.situationBus.wP.wayPointArray(49, 1).z = 0;
% y1.situationBus.wP.wayPointArray(49, 1).treach = 0;
% y1.situationBus.wP.wayPointArray(50, 1).x = 0;
% y1.situationBus.wP.wayPointArray(50, 1).y = 0;
% y1.situationBus.wP.wayPointArray(50, 1).z = 0;
% y1.situationBus.wP.wayPointArray(50, 1).treach = 0;
% y1.situationBus.wP.wayPointArray(51, 1).x = 0;
% y1.situationBus.wP.wayPointArray(51, 1).y = 0;
% y1.situationBus.wP.wayPointArray(51, 1).z = 0;
% y1.situationBus.wP.wayPointArray(51, 1).treach = 0;
% y1.situationBus.wP.wayPointArray(52, 1).x = 0;
% y1.situationBus.wP.wayPointArray(52, 1).y = 0;
% y1.situationBus.wP.wayPointArray(52, 1).z = 0;
% y1.situationBus.wP.wayPointArray(52, 1).treach = 0;
% y1.situationBus.wP.wayPointArray(53, 1).x = 0;
% y1.situationBus.wP.wayPointArray(53, 1).y = 0;
% y1.situationBus.wP.wayPointArray(53, 1).z = 0;
% y1.situationBus.wP.wayPointArray(53, 1).treach = 0;
% y1.situationBus.wP.wayPointArray(54, 1).x = 0;
% y1.situationBus.wP.wayPointArray(54, 1).y = 0;
% y1.situationBus.wP.wayPointArray(54, 1).z = 0;
% y1.situationBus.wP.wayPointArray(54, 1).treach = 0;
% y1.situationBus.wP.wayPointArray(55, 1).x = 0;
% y1.situationBus.wP.wayPointArray(55, 1).y = 0;
% y1.situationBus.wP.wayPointArray(55, 1).z = 0;
% y1.situationBus.wP.wayPointArray(55, 1).treach = 0;
% y1.situationBus.wP.wayPointArray(56, 1).x = 0;
% y1.situationBus.wP.wayPointArray(56, 1).y = 0;
% y1.situationBus.wP.wayPointArray(56, 1).z = 0;
% y1.situationBus.wP.wayPointArray(56, 1).treach = 0;
% y1.situationBus.wP.wayPointArray(57, 1).x = 0;
% y1.situationBus.wP.wayPointArray(57, 1).y = 0;
% y1.situationBus.wP.wayPointArray(57, 1).z = 0;
% y1.situationBus.wP.wayPointArray(57, 1).treach = 0;
% y1.situationBus.wP.wayPointArray(58, 1).x = 0;
% y1.situationBus.wP.wayPointArray(58, 1).y = 0;
% y1.situationBus.wP.wayPointArray(58, 1).z = 0;
% y1.situationBus.wP.wayPointArray(58, 1).treach = 0;
% y1.situationBus.wP.wayPointArray(59, 1).x = 0;
% y1.situationBus.wP.wayPointArray(59, 1).y = 0;
% y1.situationBus.wP.wayPointArray(59, 1).z = 0;
% y1.situationBus.wP.wayPointArray(59, 1).treach = 0;
% y1.situationBus.wP.wayPointArray(60, 1).x = 0;
% y1.situationBus.wP.wayPointArray(60, 1).y = 0;
% y1.situationBus.wP.wayPointArray(60, 1).z = 0;
% y1.situationBus.wP.wayPointArray(60, 1).treach = 0;
% y1.situationBus.wP.wayPointArray(61, 1).x = 0;
% y1.situationBus.wP.wayPointArray(61, 1).y = 0;
% y1.situationBus.wP.wayPointArray(61, 1).z = 0;
% y1.situationBus.wP.wayPointArray(61, 1).treach = 0;
% y1.situationBus.wP.wayPointArray(62, 1).x = 0;
% y1.situationBus.wP.wayPointArray(62, 1).y = 0;
% y1.situationBus.wP.wayPointArray(62, 1).z = 0;
% y1.situationBus.wP.wayPointArray(62, 1).treach = 0;
% y1.situationBus.wP.wayPointArray(63, 1).x = 0;
% y1.situationBus.wP.wayPointArray(63, 1).y = 0;
% y1.situationBus.wP.wayPointArray(63, 1).z = 0;
% y1.situationBus.wP.wayPointArray(63, 1).treach = 0;
% y1.situationBus.wP.wayPointArray(64, 1).x = 0;
% y1.situationBus.wP.wayPointArray(64, 1).y = 0;
% y1.situationBus.wP.wayPointArray(64, 1).z = 0;
% y1.situationBus.wP.wayPointArray(64, 1).treach = 0;
% y1.situationBus.wP.wayPointArray(65, 1).x = 0;
% y1.situationBus.wP.wayPointArray(65, 1).y = 0;
% y1.situationBus.wP.wayPointArray(65, 1).z = 0;
% y1.situationBus.wP.wayPointArray(65, 1).treach = 0;
% y1.situationBus.wP.wayPointArray(66, 1).x = 0;
% y1.situationBus.wP.wayPointArray(66, 1).y = 0;
% y1.situationBus.wP.wayPointArray(66, 1).z = 0;
% y1.situationBus.wP.wayPointArray(66, 1).treach = 0;
% y1.situationBus.wP.wayPointArray(67, 1).x = 0;
% y1.situationBus.wP.wayPointArray(67, 1).y = 0;
% y1.situationBus.wP.wayPointArray(67, 1).z = 0;
% y1.situationBus.wP.wayPointArray(67, 1).treach = 0;
% y1.situationBus.wP.wayPointArray(68, 1).x = 0;
% y1.situationBus.wP.wayPointArray(68, 1).y = 0;
% y1.situationBus.wP.wayPointArray(68, 1).z = 0;
% y1.situationBus.wP.wayPointArray(68, 1).treach = 0;
% y1.situationBus.wP.wayPointArray(69, 1).x = 0;
% y1.situationBus.wP.wayPointArray(69, 1).y = 0;
% y1.situationBus.wP.wayPointArray(69, 1).z = 0;
% y1.situationBus.wP.wayPointArray(69, 1).treach = 0;
% y1.situationBus.wP.wayPointArray(70, 1).x = 0;
% y1.situationBus.wP.wayPointArray(70, 1).y = 0;
% y1.situationBus.wP.wayPointArray(70, 1).z = 0;
% y1.situationBus.wP.wayPointArray(70, 1).treach = 0;
% y1.situationBus.wP.wayPointArray(71, 1).x = 0;
% y1.situationBus.wP.wayPointArray(71, 1).y = 0;
% y1.situationBus.wP.wayPointArray(71, 1).z = 0;
% y1.situationBus.wP.wayPointArray(71, 1).treach = 0;
% y1.situationBus.wP.wayPointArray(72, 1).x = 0;
% y1.situationBus.wP.wayPointArray(72, 1).y = 0;
% y1.situationBus.wP.wayPointArray(72, 1).z = 0;
% y1.situationBus.wP.wayPointArray(72, 1).treach = 0;
% y1.situationBus.wP.wayPointArray(73, 1).x = 0;
% y1.situationBus.wP.wayPointArray(73, 1).y = 0;
% y1.situationBus.wP.wayPointArray(73, 1).z = 0;
% y1.situationBus.wP.wayPointArray(73, 1).treach = 0;
% y1.situationBus.wP.wayPointArray(74, 1).x = 0;
% y1.situationBus.wP.wayPointArray(74, 1).y = 0;
% y1.situationBus.wP.wayPointArray(74, 1).z = 0;
% y1.situationBus.wP.wayPointArray(74, 1).treach = 0;
% y1.situationBus.wP.wayPointArray(75, 1).x = 0;
% y1.situationBus.wP.wayPointArray(75, 1).y = 0;
% y1.situationBus.wP.wayPointArray(75, 1).z = 0;
% y1.situationBus.wP.wayPointArray(75, 1).treach = 0;
% y1.situationBus.wP.wayPointArray(76, 1).x = 0;
% y1.situationBus.wP.wayPointArray(76, 1).y = 0;
% y1.situationBus.wP.wayPointArray(76, 1).z = 0;
% y1.situationBus.wP.wayPointArray(76, 1).treach = 0;
% y1.situationBus.wP.wayPointArray(77, 1).x = 0;
% y1.situationBus.wP.wayPointArray(77, 1).y = 0;
% y1.situationBus.wP.wayPointArray(77, 1).z = 0;
% y1.situationBus.wP.wayPointArray(77, 1).treach = 0;
% y1.situationBus.wP.wayPointArray(78, 1).x = 0;
% y1.situationBus.wP.wayPointArray(78, 1).y = 0;
% y1.situationBus.wP.wayPointArray(78, 1).z = 0;
% y1.situationBus.wP.wayPointArray(78, 1).treach = 0;
% y1.situationBus.wP.wayPointArray(79, 1).x = 0;
% y1.situationBus.wP.wayPointArray(79, 1).y = 0;
% y1.situationBus.wP.wayPointArray(79, 1).z = 0;
% y1.situationBus.wP.wayPointArray(79, 1).treach = 0;
% y1.situationBus.wP.wayPointArray(80, 1).x = 0;
% y1.situationBus.wP.wayPointArray(80, 1).y = 0;
% y1.situationBus.wP.wayPointArray(80, 1).z = 0;
% y1.situationBus.wP.wayPointArray(80, 1).treach = 0;
% y1.situationBus.wP.wayPointArray(81, 1).x = 0;
% y1.situationBus.wP.wayPointArray(81, 1).y = 0;
% y1.situationBus.wP.wayPointArray(81, 1).z = 0;
% y1.situationBus.wP.wayPointArray(81, 1).treach = 0;
% y1.situationBus.wP.wayPointArray(82, 1).x = 0;
% y1.situationBus.wP.wayPointArray(82, 1).y = 0;
% y1.situationBus.wP.wayPointArray(82, 1).z = 0;
% y1.situationBus.wP.wayPointArray(82, 1).treach = 0;
% y1.situationBus.wP.wayPointArray(83, 1).x = 0;
% y1.situationBus.wP.wayPointArray(83, 1).y = 0;
% y1.situationBus.wP.wayPointArray(83, 1).z = 0;
% y1.situationBus.wP.wayPointArray(83, 1).treach = 0;
% y1.situationBus.wP.wayPointArray(84, 1).x = 0;
% y1.situationBus.wP.wayPointArray(84, 1).y = 0;
% y1.situationBus.wP.wayPointArray(84, 1).z = 0;
% y1.situationBus.wP.wayPointArray(84, 1).treach = 0;
% y1.situationBus.wP.wayPointArray(85, 1).x = 0;
% y1.situationBus.wP.wayPointArray(85, 1).y = 0;
% y1.situationBus.wP.wayPointArray(85, 1).z = 0;
% y1.situationBus.wP.wayPointArray(85, 1).treach = 0;
% y1.situationBus.wP.wayPointArray(86, 1).x = 0;
% y1.situationBus.wP.wayPointArray(86, 1).y = 0;
% y1.situationBus.wP.wayPointArray(86, 1).z = 0;
% y1.situationBus.wP.wayPointArray(86, 1).treach = 0;
% y1.situationBus.wP.wayPointArray(87, 1).x = 0;
% y1.situationBus.wP.wayPointArray(87, 1).y = 0;
% y1.situationBus.wP.wayPointArray(87, 1).z = 0;
% y1.situationBus.wP.wayPointArray(87, 1).treach = 0;
% y1.situationBus.wP.wayPointArray(88, 1).x = 0;
% y1.situationBus.wP.wayPointArray(88, 1).y = 0;
% y1.situationBus.wP.wayPointArray(88, 1).z = 0;
% y1.situationBus.wP.wayPointArray(88, 1).treach = 0;
% y1.situationBus.wP.wayPointArray(89, 1).x = 0;
% y1.situationBus.wP.wayPointArray(89, 1).y = 0;
% y1.situationBus.wP.wayPointArray(89, 1).z = 0;
% y1.situationBus.wP.wayPointArray(89, 1).treach = 0;
% y1.situationBus.wP.wayPointArray(90, 1).x = 0;
% y1.situationBus.wP.wayPointArray(90, 1).y = 0;
% y1.situationBus.wP.wayPointArray(90, 1).z = 0;
% y1.situationBus.wP.wayPointArray(90, 1).treach = 0;
% y1.situationBus.wP.wayPointArray(91, 1).x = 0;
% y1.situationBus.wP.wayPointArray(91, 1).y = 0;
% y1.situationBus.wP.wayPointArray(91, 1).z = 0;
% y1.situationBus.wP.wayPointArray(91, 1).treach = 0;
% y1.situationBus.wP.wayPointArray(92, 1).x = 0;
% y1.situationBus.wP.wayPointArray(92, 1).y = 0;
% y1.situationBus.wP.wayPointArray(92, 1).z = 0;
% y1.situationBus.wP.wayPointArray(92, 1).treach = 0;
% y1.situationBus.wP.wayPointArray(93, 1).x = 0;
% y1.situationBus.wP.wayPointArray(93, 1).y = 0;
% y1.situationBus.wP.wayPointArray(93, 1).z = 0;
% y1.situationBus.wP.wayPointArray(93, 1).treach = 0;
% y1.situationBus.wP.wayPointArray(94, 1).x = 0;
% y1.situationBus.wP.wayPointArray(94, 1).y = 0;
% y1.situationBus.wP.wayPointArray(94, 1).z = 0;
% y1.situationBus.wP.wayPointArray(94, 1).treach = 0;
% y1.situationBus.wP.wayPointArray(95, 1).x = 0;
% y1.situationBus.wP.wayPointArray(95, 1).y = 0;
% y1.situationBus.wP.wayPointArray(95, 1).z = 0;
% y1.situationBus.wP.wayPointArray(95, 1).treach = 0;
% y1.situationBus.wP.wayPointArray(96, 1).x = 0;
% y1.situationBus.wP.wayPointArray(96, 1).y = 0;
% y1.situationBus.wP.wayPointArray(96, 1).z = 0;
% y1.situationBus.wP.wayPointArray(96, 1).treach = 0;
% y1.situationBus.wP.wayPointArray(97, 1).x = 0;
% y1.situationBus.wP.wayPointArray(97, 1).y = 0;
% y1.situationBus.wP.wayPointArray(97, 1).z = 0;
% y1.situationBus.wP.wayPointArray(97, 1).treach = 0;
% y1.situationBus.wP.wayPointArray(98, 1).x = 0;
% y1.situationBus.wP.wayPointArray(98, 1).y = 0;
% y1.situationBus.wP.wayPointArray(98, 1).z = 0;
% y1.situationBus.wP.wayPointArray(98, 1).treach = 0;
% y1.situationBus.wP.wayPointArray(99, 1).x = 0;
% y1.situationBus.wP.wayPointArray(99, 1).y = 0;
% y1.situationBus.wP.wayPointArray(99, 1).z = 0;
% y1.situationBus.wP.wayPointArray(99, 1).treach = 0;
% y1.situationBus.wP.wayPointArray(100, 1).x = 0;
% y1.situationBus.wP.wayPointArray(100, 1).y = 0;
% y1.situationBus.wP.wayPointArray(100, 1).z = 0;
% y1.situationBus.wP.wayPointArray(100, 1).treach = 0;
% 
% y1.situationBus.selfAwarenessBus.x = 0;
% y1.situationBus.selfAwarenessBus.y = 0;
% y1.situationBus.selfAwarenessBus.z = 0;
% y1.situationBus.selfAwarenessBus.theta = 0;
% y1.situationBus.selfAwarenessBus.phi = 0;
% y1.situationBus.selfAwarenessBus.psi = 0;
% y1.situationBus.selfAwarenessBus.u = 0;
% y1.situationBus.selfAwarenessBus.v = 0;
% y1.situationBus.selfAwarenessBus.w = 0;
% y1.situationBus.selfAwarenessBus.dtheta = 0;
% y1.situationBus.selfAwarenessBus.dphi = 0;
% y1.situationBus.selfAwarenessBus.dpsi = 0;
% y1.IdealSensors = struct;
% y1.IdealSensors.x = 0;
% y1.IdealSensors.y = 0;
% y1.IdealSensors.z = 0;
% y1.IdealSensors.theta = 0;
% y1.IdealSensors.phi = 0;
% y1.IdealSensors.psi = 0;
% y1.IdealSensors.u = 0;
% y1.IdealSensors.v = 0;
% y1.IdealSensors.w = 0;
% y1.IdealSensors.dtheta = 0;
% y1.IdealSensors.dphi = 0;
% y1.IdealSensors.dpsi = 0;
% y1.FromPrescan = struct;
% y1.FromPrescan.x = 0;
% y1.FromPrescan.y = 0;
% y1.FromPrescan.z = 0;
% y1.FromPrescan.Rotx = 0;
% y1.FromPrescan.Roty = 0;
% y1.FromPrescan.Rotz = 0;
% y1.FromPrescan.GPS_lat = 0;
% y1.FromPrescan.GPS_long = 0;
% y1.FromPrescan.u = 0;
% y1.FromPrescan.GPS_alt = 0;
% y1.FromPrescan.heading = 0;
% y1.FromPrescan.Yaw_rate = 0;
% y1.ConnectedBus = struct;
% y1.ConnectedBus.ObjectsBus = struct;
% y1.ConnectedBus.ObjectsBus(1, 1).x = 0;
% y1.ConnectedBus.ObjectsBus(1, 1).y = 0;
% y1.ConnectedBus.ObjectsBus(1, 1).yaw = 0;
% y1.ConnectedBus.ObjectsBus(2, 1).x = 0;
% y1.ConnectedBus.ObjectsBus(2, 1).y = 0;
% y1.ConnectedBus.ObjectsBus(2, 1).yaw = 0;
% y1.ConnectedBus.ObjectsBus(3, 1).x = 0;
% y1.ConnectedBus.ObjectsBus(3, 1).y = 0;
% y1.ConnectedBus.ObjectsBus(3, 1).yaw = 0;
% y1.ConnectedBus.ObjectsBus(4, 1).x = 0;
% y1.ConnectedBus.ObjectsBus(4, 1).y = 0;
% y1.ConnectedBus.ObjectsBus(4, 1).yaw = 0;
% y1.ConnectedBus.ObjectsBus(5, 1).x = 0;
% y1.ConnectedBus.ObjectsBus(5, 1).y = 0;
% y1.ConnectedBus.ObjectsBus(5, 1).yaw = 0;
% y1.ConnectedBus.ObjectsBus(6, 1).x = 0;
% y1.ConnectedBus.ObjectsBus(6, 1).y = 0;
% y1.ConnectedBus.ObjectsBus(6, 1).yaw = 0;
% y1.ConnectedBus.ObjectsBus(7, 1).x = 0;
% y1.ConnectedBus.ObjectsBus(7, 1).y = 0;
% y1.ConnectedBus.ObjectsBus(7, 1).yaw = 0;
% y1.ConnectedBus.ObjectsBus(8, 1).x = 0;
% y1.ConnectedBus.ObjectsBus(8, 1).y = 0;
% y1.ConnectedBus.ObjectsBus(8, 1).yaw = 0;
% y1.ConnectedBus.ObjectsBus(9, 1).x = 0;
% y1.ConnectedBus.ObjectsBus(9, 1).y = 0;
% y1.ConnectedBus.ObjectsBus(9, 1).yaw = 0;
% y1.ConnectedBus.ObjectsBus(10, 1).x = 0;
% y1.ConnectedBus.ObjectsBus(10, 1).y = 0;
% y1.ConnectedBus.ObjectsBus(10, 1).yaw = 0;
% y1.ConnectedBus.ObjectsBus(11, 1).x = 0;
% y1.ConnectedBus.ObjectsBus(11, 1).y = 0;
% y1.ConnectedBus.ObjectsBus(11, 1).yaw = 0;
% y1.ConnectedBus.ObjectsBus(12, 1).x = 0;
% y1.ConnectedBus.ObjectsBus(12, 1).y = 0;
% y1.ConnectedBus.ObjectsBus(12, 1).yaw = 0;
% y1.ConnectedBus.ObjectsBus(13, 1).x = 0;
% y1.ConnectedBus.ObjectsBus(13, 1).y = 0;
% y1.ConnectedBus.ObjectsBus(13, 1).yaw = 0;
% y1.ConnectedBus.ObjectsBus(14, 1).x = 0;
% y1.ConnectedBus.ObjectsBus(14, 1).y = 0;
% y1.ConnectedBus.ObjectsBus(14, 1).yaw = 0;
% y1.ConnectedBus.ObjectsBus(15, 1).x = 0;
% y1.ConnectedBus.ObjectsBus(15, 1).y = 0;
% y1.ConnectedBus.ObjectsBus(15, 1).yaw = 0;
% y1.ConnectedBus.ObjectsBus(16, 1).x = 0;
% y1.ConnectedBus.ObjectsBus(16, 1).y = 0;
% y1.ConnectedBus.ObjectsBus(16, 1).yaw = 0;
% y1.ConnectedBus.ObjectsBus(17, 1).x = 0;
% y1.ConnectedBus.ObjectsBus(17, 1).y = 0;
% y1.ConnectedBus.ObjectsBus(17, 1).yaw = 0;
% y1.ConnectedBus.ObjectsBus(18, 1).x = 0;
% y1.ConnectedBus.ObjectsBus(18, 1).y = 0;
% y1.ConnectedBus.ObjectsBus(18, 1).yaw = 0;
% y1.ConnectedBus.ObjectsBus(19, 1).x = 0;
% y1.ConnectedBus.ObjectsBus(19, 1).y = 0;
% y1.ConnectedBus.ObjectsBus(19, 1).yaw = 0;
% y1.ConnectedBus.ObjectsBus(20, 1).x = 0;
% y1.ConnectedBus.ObjectsBus(20, 1).y = 0;
% y1.ConnectedBus.ObjectsBus(20, 1).yaw = 0;
% y1.ConnectedBus.ObjectsBus(21, 1).x = 0;
% y1.ConnectedBus.ObjectsBus(21, 1).y = 0;
% y1.ConnectedBus.ObjectsBus(21, 1).yaw = 0;
% y1.ConnectedBus.ObjectsBus(22, 1).x = 0;
% y1.ConnectedBus.ObjectsBus(22, 1).y = 0;
% y1.ConnectedBus.ObjectsBus(22, 1).yaw = 0;
% y1.ConnectedBus.ObjectsBus(23, 1).x = 0;
% y1.ConnectedBus.ObjectsBus(23, 1).y = 0;
% y1.ConnectedBus.ObjectsBus(23, 1).yaw = 0;
% y1.ConnectedBus.ObjectsBus(24, 1).x = 0;
% y1.ConnectedBus.ObjectsBus(24, 1).y = 0;
% y1.ConnectedBus.ObjectsBus(24, 1).yaw = 0;
% y1.ConnectedBus.ObjectsBus(25, 1).x = 0;
% y1.ConnectedBus.ObjectsBus(25, 1).y = 0;
% y1.ConnectedBus.ObjectsBus(25, 1).yaw = 0;
% y1.ConnectedBus.ObjectsBus(26, 1).x = 0;
% y1.ConnectedBus.ObjectsBus(26, 1).y = 0;
% y1.ConnectedBus.ObjectsBus(26, 1).yaw = 0;
% y1.ConnectedBus.ObjectsBus(27, 1).x = 0;
% y1.ConnectedBus.ObjectsBus(27, 1).y = 0;
% y1.ConnectedBus.ObjectsBus(27, 1).yaw = 0;
% y1.ConnectedBus.ObjectsBus(28, 1).x = 0;
% y1.ConnectedBus.ObjectsBus(28, 1).y = 0;
% y1.ConnectedBus.ObjectsBus(28, 1).yaw = 0;
% y1.ConnectedBus.ObjectsBus(29, 1).x = 0;
% y1.ConnectedBus.ObjectsBus(29, 1).y = 0;
% y1.ConnectedBus.ObjectsBus(29, 1).yaw = 0;
% y1.ConnectedBus.ObjectsBus(30, 1).x = 0;
% y1.ConnectedBus.ObjectsBus(30, 1).y = 0;
% y1.ConnectedBus.ObjectsBus(30, 1).yaw = 0;
% y1.ConnectedBus.ObjectsBus(31, 1).x = 0;
% y1.ConnectedBus.ObjectsBus(31, 1).y = 0;
% y1.ConnectedBus.ObjectsBus(31, 1).yaw = 0;
% y1.ConnectedBus.ObjectsBus(32, 1).x = 0;
% y1.ConnectedBus.ObjectsBus(32, 1).y = 0;
% y1.ConnectedBus.ObjectsBus(32, 1).yaw = 0;
% y1.ConnectedBus.ObjectsBus(33, 1).x = 0;
% y1.ConnectedBus.ObjectsBus(33, 1).y = 0;
% y1.ConnectedBus.ObjectsBus(33, 1).yaw = 0;
% y1.ConnectedBus.ObjectsBus(34, 1).x = 0;
% y1.ConnectedBus.ObjectsBus(34, 1).y = 0;
% y1.ConnectedBus.ObjectsBus(34, 1).yaw = 0;
% y1.ConnectedBus.ObjectsBus(35, 1).x = 0;
% y1.ConnectedBus.ObjectsBus(35, 1).y = 0;
% y1.ConnectedBus.ObjectsBus(35, 1).yaw = 0;
% y1.ConnectedBus.ObjectsBus(36, 1).x = 0;
% y1.ConnectedBus.ObjectsBus(36, 1).y = 0;
% y1.ConnectedBus.ObjectsBus(36, 1).yaw = 0;
% y1.ConnectedBus.ObjectsBus(37, 1).x = 0;
% y1.ConnectedBus.ObjectsBus(37, 1).y = 0;
% y1.ConnectedBus.ObjectsBus(37, 1).yaw = 0;
% y1.ConnectedBus.ObjectsBus(38, 1).x = 0;
% y1.ConnectedBus.ObjectsBus(38, 1).y = 0;
% y1.ConnectedBus.ObjectsBus(38, 1).yaw = 0;
% y1.ConnectedBus.ObjectsBus(39, 1).x = 0;
% y1.ConnectedBus.ObjectsBus(39, 1).y = 0;
% y1.ConnectedBus.ObjectsBus(39, 1).yaw = 0;
% y1.ConnectedBus.ObjectsBus(40, 1).x = 0;
% y1.ConnectedBus.ObjectsBus(40, 1).y = 0;
% y1.ConnectedBus.ObjectsBus(40, 1).yaw = 0;
% y1.ConnectedBus.ObjectsBus(41, 1).x = 0;
% y1.ConnectedBus.ObjectsBus(41, 1).y = 0;
% y1.ConnectedBus.ObjectsBus(41, 1).yaw = 0;
% y1.ConnectedBus.ObjectsBus(42, 1).x = 0;
% y1.ConnectedBus.ObjectsBus(42, 1).y = 0;
% y1.ConnectedBus.ObjectsBus(42, 1).yaw = 0;
% y1.ConnectedBus.ObjectsBus(43, 1).x = 0;
% y1.ConnectedBus.ObjectsBus(43, 1).y = 0;
% y1.ConnectedBus.ObjectsBus(43, 1).yaw = 0;
% y1.ConnectedBus.ObjectsBus(44, 1).x = 0;
% y1.ConnectedBus.ObjectsBus(44, 1).y = 0;
% y1.ConnectedBus.ObjectsBus(44, 1).yaw = 0;
% y1.ConnectedBus.ObjectsBus(45, 1).x = 0;
% y1.ConnectedBus.ObjectsBus(45, 1).y = 0;
% y1.ConnectedBus.ObjectsBus(45, 1).yaw = 0;
% y1.ConnectedBus.ObjectsBus(46, 1).x = 0;
% y1.ConnectedBus.ObjectsBus(46, 1).y = 0;
% y1.ConnectedBus.ObjectsBus(46, 1).yaw = 0;
% y1.ConnectedBus.ObjectsBus(47, 1).x = 0;
% y1.ConnectedBus.ObjectsBus(47, 1).y = 0;
% y1.ConnectedBus.ObjectsBus(47, 1).yaw = 0;
% y1.ConnectedBus.ObjectsBus(48, 1).x = 0;
% y1.ConnectedBus.ObjectsBus(48, 1).y = 0;
% y1.ConnectedBus.ObjectsBus(48, 1).yaw = 0;
% y1.ConnectedBus.ObjectsBus(49, 1).x = 0;
% y1.ConnectedBus.ObjectsBus(49, 1).y = 0;
% y1.ConnectedBus.ObjectsBus(49, 1).yaw = 0;
% y1.ConnectedBus.ObjectsBus(50, 1).x = 0;
% y1.ConnectedBus.ObjectsBus(50, 1).y = 0;
% y1.ConnectedBus.ObjectsBus(50, 1).yaw = 0;
% y1.ConnectedBus.ObjectsBus(51, 1).x = 0;
% y1.ConnectedBus.ObjectsBus(51, 1).y = 0;
% y1.ConnectedBus.ObjectsBus(51, 1).yaw = 0;
% y1.ConnectedBus.ObjectsBus(52, 1).x = 0;
% y1.ConnectedBus.ObjectsBus(52, 1).y = 0;
% y1.ConnectedBus.ObjectsBus(52, 1).yaw = 0;
% y1.ConnectedBus.ObjectsBus(53, 1).x = 0;
% y1.ConnectedBus.ObjectsBus(53, 1).y = 0;
% y1.ConnectedBus.ObjectsBus(53, 1).yaw = 0;
% y1.ConnectedBus.ObjectsBus(54, 1).x = 0;
% y1.ConnectedBus.ObjectsBus(54, 1).y = 0;
% y1.ConnectedBus.ObjectsBus(54, 1).yaw = 0;
% y1.ConnectedBus.ObjectsBus(55, 1).x = 0;
% y1.ConnectedBus.ObjectsBus(55, 1).y = 0;
% y1.ConnectedBus.ObjectsBus(55, 1).yaw = 0;
% y1.ConnectedBus.ObjectsBus(56, 1).x = 0;
% y1.ConnectedBus.ObjectsBus(56, 1).y = 0;
% y1.ConnectedBus.ObjectsBus(56, 1).yaw = 0;
% y1.ConnectedBus.ObjectsBus(57, 1).x = 0;
% y1.ConnectedBus.ObjectsBus(57, 1).y = 0;
% y1.ConnectedBus.ObjectsBus(57, 1).yaw = 0;
% y1.ConnectedBus.ObjectsBus(58, 1).x = 0;
% y1.ConnectedBus.ObjectsBus(58, 1).y = 0;
% y1.ConnectedBus.ObjectsBus(58, 1).yaw = 0;
% y1.ConnectedBus.ObjectsBus(59, 1).x = 0;
% y1.ConnectedBus.ObjectsBus(59, 1).y = 0;
% y1.ConnectedBus.ObjectsBus(59, 1).yaw = 0;
% y1.ConnectedBus.ObjectsBus(60, 1).x = 0;
% y1.ConnectedBus.ObjectsBus(60, 1).y = 0;
% y1.ConnectedBus.ObjectsBus(60, 1).yaw = 0;
% y1.ConnectedBus.ObjectsBus(61, 1).x = 0;
% y1.ConnectedBus.ObjectsBus(61, 1).y = 0;
% y1.ConnectedBus.ObjectsBus(61, 1).yaw = 0;
% y1.ConnectedBus.ObjectsBus(62, 1).x = 0;
% y1.ConnectedBus.ObjectsBus(62, 1).y = 0;
% y1.ConnectedBus.ObjectsBus(62, 1).yaw = 0;
% y1.ConnectedBus.ObjectsBus(63, 1).x = 0;
% y1.ConnectedBus.ObjectsBus(63, 1).y = 0;
% y1.ConnectedBus.ObjectsBus(63, 1).yaw = 0;
% y1.ConnectedBus.ObjectsBus(64, 1).x = 0;
% y1.ConnectedBus.ObjectsBus(64, 1).y = 0;
% y1.ConnectedBus.ObjectsBus(64, 1).yaw = 0;
% y1.ConnectedBus.ObjectsBus(65, 1).x = 0;
% y1.ConnectedBus.ObjectsBus(65, 1).y = 0;
% y1.ConnectedBus.ObjectsBus(65, 1).yaw = 0;
% y1.ConnectedBus.ObjectsBus(66, 1).x = 0;
% y1.ConnectedBus.ObjectsBus(66, 1).y = 0;
% y1.ConnectedBus.ObjectsBus(66, 1).yaw = 0;
% y1.ConnectedBus.ObjectsBus(67, 1).x = 0;
% y1.ConnectedBus.ObjectsBus(67, 1).y = 0;
% y1.ConnectedBus.ObjectsBus(67, 1).yaw = 0;
% y1.ConnectedBus.ObjectsBus(68, 1).x = 0;
% y1.ConnectedBus.ObjectsBus(68, 1).y = 0;
% y1.ConnectedBus.ObjectsBus(68, 1).yaw = 0;
% y1.ConnectedBus.ObjectsBus(69, 1).x = 0;
% y1.ConnectedBus.ObjectsBus(69, 1).y = 0;
% y1.ConnectedBus.ObjectsBus(69, 1).yaw = 0;
% y1.ConnectedBus.ObjectsBus(70, 1).x = 0;
% y1.ConnectedBus.ObjectsBus(70, 1).y = 0;
% y1.ConnectedBus.ObjectsBus(70, 1).yaw = 0;
% y1.ConnectedBus.ObjectsBus(71, 1).x = 0;
% y1.ConnectedBus.ObjectsBus(71, 1).y = 0;
% y1.ConnectedBus.ObjectsBus(71, 1).yaw = 0;
% y1.ConnectedBus.ObjectsBus(72, 1).x = 0;
% y1.ConnectedBus.ObjectsBus(72, 1).y = 0;
% y1.ConnectedBus.ObjectsBus(72, 1).yaw = 0;
% y1.ConnectedBus.ObjectsBus(73, 1).x = 0;
% y1.ConnectedBus.ObjectsBus(73, 1).y = 0;
% y1.ConnectedBus.ObjectsBus(73, 1).yaw = 0;
% y1.ConnectedBus.ObjectsBus(74, 1).x = 0;
% y1.ConnectedBus.ObjectsBus(74, 1).y = 0;
% y1.ConnectedBus.ObjectsBus(74, 1).yaw = 0;
% y1.ConnectedBus.ObjectsBus(75, 1).x = 0;
% y1.ConnectedBus.ObjectsBus(75, 1).y = 0;
% y1.ConnectedBus.ObjectsBus(75, 1).yaw = 0;
% y1.ConnectedBus.ObjectsBus(76, 1).x = 0;
% y1.ConnectedBus.ObjectsBus(76, 1).y = 0;
% y1.ConnectedBus.ObjectsBus(76, 1).yaw = 0;
% y1.ConnectedBus.ObjectsBus(77, 1).x = 0;
% y1.ConnectedBus.ObjectsBus(77, 1).y = 0;
% y1.ConnectedBus.ObjectsBus(77, 1).yaw = 0;
% y1.ConnectedBus.ObjectsBus(78, 1).x = 0;
% y1.ConnectedBus.ObjectsBus(78, 1).y = 0;
% y1.ConnectedBus.ObjectsBus(78, 1).yaw = 0;
% y1.ConnectedBus.ObjectsBus(79, 1).x = 0;
% y1.ConnectedBus.ObjectsBus(79, 1).y = 0;
% y1.ConnectedBus.ObjectsBus(79, 1).yaw = 0;
% y1.ConnectedBus.ObjectsBus(80, 1).x = 0;
% y1.ConnectedBus.ObjectsBus(80, 1).y = 0;
% y1.ConnectedBus.ObjectsBus(80, 1).yaw = 0;
% y1.ConnectedBus.ObjectsBus(81, 1).x = 0;
% y1.ConnectedBus.ObjectsBus(81, 1).y = 0;
% y1.ConnectedBus.ObjectsBus(81, 1).yaw = 0;
% y1.ConnectedBus.ObjectsBus(82, 1).x = 0;
% y1.ConnectedBus.ObjectsBus(82, 1).y = 0;
% y1.ConnectedBus.ObjectsBus(82, 1).yaw = 0;
% y1.ConnectedBus.ObjectsBus(83, 1).x = 0;
% y1.ConnectedBus.ObjectsBus(83, 1).y = 0;
% y1.ConnectedBus.ObjectsBus(83, 1).yaw = 0;
% y1.ConnectedBus.ObjectsBus(84, 1).x = 0;
% y1.ConnectedBus.ObjectsBus(84, 1).y = 0;
% y1.ConnectedBus.ObjectsBus(84, 1).yaw = 0;
% y1.ConnectedBus.ObjectsBus(85, 1).x = 0;
% y1.ConnectedBus.ObjectsBus(85, 1).y = 0;
% y1.ConnectedBus.ObjectsBus(85, 1).yaw = 0;
% y1.ConnectedBus.ObjectsBus(86, 1).x = 0;
% y1.ConnectedBus.ObjectsBus(86, 1).y = 0;
% y1.ConnectedBus.ObjectsBus(86, 1).yaw = 0;
% y1.ConnectedBus.ObjectsBus(87, 1).x = 0;
% y1.ConnectedBus.ObjectsBus(87, 1).y = 0;
% y1.ConnectedBus.ObjectsBus(87, 1).yaw = 0;
% y1.ConnectedBus.ObjectsBus(88, 1).x = 0;
% y1.ConnectedBus.ObjectsBus(88, 1).y = 0;
% y1.ConnectedBus.ObjectsBus(88, 1).yaw = 0;
% y1.ConnectedBus.ObjectsBus(89, 1).x = 0;
% y1.ConnectedBus.ObjectsBus(89, 1).y = 0;
% y1.ConnectedBus.ObjectsBus(89, 1).yaw = 0;
% y1.ConnectedBus.ObjectsBus(90, 1).x = 0;
% y1.ConnectedBus.ObjectsBus(90, 1).y = 0;
% y1.ConnectedBus.ObjectsBus(90, 1).yaw = 0;
% y1.ConnectedBus.ObjectsBus(91, 1).x = 0;
% y1.ConnectedBus.ObjectsBus(91, 1).y = 0;
% y1.ConnectedBus.ObjectsBus(91, 1).yaw = 0;
% y1.ConnectedBus.ObjectsBus(92, 1).x = 0;
% y1.ConnectedBus.ObjectsBus(92, 1).y = 0;
% y1.ConnectedBus.ObjectsBus(92, 1).yaw = 0;
% y1.ConnectedBus.ObjectsBus(93, 1).x = 0;
% y1.ConnectedBus.ObjectsBus(93, 1).y = 0;
% y1.ConnectedBus.ObjectsBus(93, 1).yaw = 0;
% y1.ConnectedBus.ObjectsBus(94, 1).x = 0;
% y1.ConnectedBus.ObjectsBus(94, 1).y = 0;
% y1.ConnectedBus.ObjectsBus(94, 1).yaw = 0;
% y1.ConnectedBus.ObjectsBus(95, 1).x = 0;
% y1.ConnectedBus.ObjectsBus(95, 1).y = 0;
% y1.ConnectedBus.ObjectsBus(95, 1).yaw = 0;
% y1.ConnectedBus.ObjectsBus(96, 1).x = 0;
% y1.ConnectedBus.ObjectsBus(96, 1).y = 0;
% y1.ConnectedBus.ObjectsBus(96, 1).yaw = 0;
% y1.ConnectedBus.ObjectsBus(97, 1).x = 0;
% y1.ConnectedBus.ObjectsBus(97, 1).y = 0;
% y1.ConnectedBus.ObjectsBus(97, 1).yaw = 0;
% y1.ConnectedBus.ObjectsBus(98, 1).x = 0;
% y1.ConnectedBus.ObjectsBus(98, 1).y = 0;
% y1.ConnectedBus.ObjectsBus(98, 1).yaw = 0;
% y1.ConnectedBus.ObjectsBus(99, 1).x = 0;
% y1.ConnectedBus.ObjectsBus(99, 1).y = 0;
% y1.ConnectedBus.ObjectsBus(99, 1).yaw = 0;
% y1.ConnectedBus.ObjectsBus(100, 1).x = 0;
% y1.ConnectedBus.ObjectsBus(100, 1).y = 0;
% y1.ConnectedBus.ObjectsBus(100, 1).yaw = 0;
% y1.ConnectedBus.NumberObjects = 0;
% 


if isempty(a)
    a = 1;
    y = y0;
    y.situationBus.wP.wayPointArray = veh_struct.initialWayPointsArray;
    y.situationBus.wP.currentWayPointIndex = veh_struct.initialCurrentWayPointIndex;
    y.situationBus.wP.finalWayPointIndex = veh_struct.initialFinalWayPointIndex;

else
    y = u;
end
